simulink library "DriftControllerLibrary"  (R2014a)
settings: Solver=ode45  StartTime=0.0  StopTime=10.0  RelTol=1e-3
values from neighbouring files (symbols this model uses):
  alpha_lookup = alpha_sl:-0.001:-1*alpha_sl    [Fyf_lookup_table.m]
  alpha_prm = 0.9    [InitMap.m]
  beta_prm = 1    [InitMap.m]
  curve_prm = curve_prm.data    [InitMap.m]
  discrete_prm = discrete_prm.data    [InitMap.m]
  errLim_prm = 0.005    [InitMap.m]
  Fyf_lookup_2W = -Cf*tan(alpha_lookup) + Cf^2*(2 - mu_s_assumed_f/mu_p_assumed_f)*abs(tan(alpha_lookup)).*tan(alpha_lookup)/(3*mu_p_assumed_f*Fzf) -      Cf^3*tan(alpha_lookup).^3*(1-2*mu_s_assumed_f/(3*mu_p_assumed_f))/(9*mu_p_assumed_f^2*Fzf^2)    [Fyf_lookup_table.m]
  Fyf_lookup_4W = -(Cf/2)*tan(alpha_lookup) + (Cf/2)^2*(2 - mu_s_assumed_f/mu_p_assumed_f)*abs(tan(alpha_lookup)).*tan(alpha_lookup)/(3*mu_p_assumed_f*(Fzf/2)) -      (Cf/2)^3*tan(alpha_lookup).^3*(1-2*mu_s_assumed_f/(3*mu_p_assumed_f))/(9*mu_p_assumed_f^2*(Fzf/2)^2)    [Fyf_lookup_table.m]
  iterLim_prm = 30    [InitMap.m]
  map_prm = map_prm.data    [InitMap.m]
  numTerms_prm = 10    [InitMap.m]
  seg_prm = seg_prm.data    [InitMap.m]
  Ts = 0.002    [DSC_Control_Analysis.m]    (also in DSC_Control_Analysis_Exp.m; DSC_Speed_Control_Analysis.m; EC_params_nissan.m; Ext_MPCPara.m = SSD.Ts)
  useZ_prm = 0    [InitMap.m]
undefined symbols (not defined in the file or in its folder): ack, axInit, beta_vec, betaDes, betaThreshold, delta_sol, deltaLimits, Feasible, Fxr_sol, FxrEq, Fyf_sat, Fyf_sol, Kbeta, Kr, KUx, KUx_Drift, mu_p_assumed, mu_s_assumed, param, r_vec, rThreshold, sr, steering_limit, tau_DK, tau_DSC, tHold, tLimits, Ux_vec, UxEq, UxLimits, VoltsToTorque, VoltsToTorqueRegen, wc
libraries: DriftControllerLibrary x2, simulink x1
(part 2 of 2)

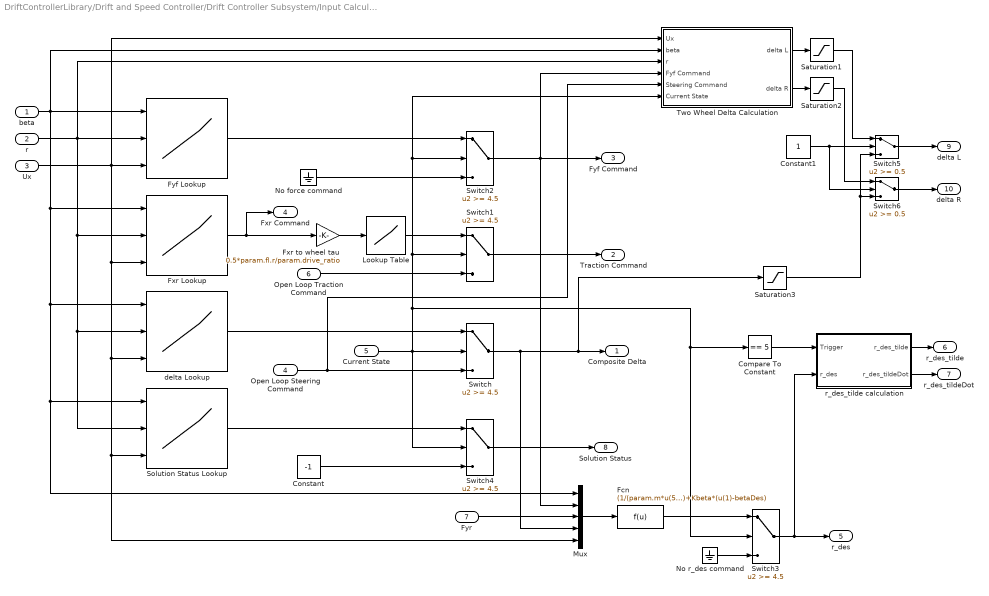
== system DriftControllerLibrary/Drift and Speed Controller/Drift Controller Subsystem/Input Calculation ==
  beta : Inport
  r : Inport  Port=2
  Ux : Inport  Port=3
  Open Loop Steering Command : Inport  Port=4
  Current State : Inport  Port=5
  Open Loop Traction Command : Inport  Port=6
  Fyr : Inport  Port=7
  Compare To Constant : simulink/Logic and Bit Operations/Compare To Constant  relop===  const=5  OutDataTypeStr=uint8  ZeroCross=off
  Constant : Constant  Value=-1
  Constant1 : Constant
  Fcn : Fcn  Expr=(1/(param.m*u(5)))*(u(2)*cos(u(4)) + u(3))+Kbeta*(u(1)-betaDes)
  Fxr Lookup : Lookup_n-D  NumberOfTableDimensions=3  BreakpointsForDimension1=beta_vec  BreakpointsForDimension2=r_vec  BreakpointsForDimension3=Ux_vec  IndexSearchMethod=Evenly spaced points  Table=Fxr_sol  ExtrapMethod=Clip  UseLastTableValue=on  InputSameDT=on
  Fxr to wheel tau : Gain  Gain=0.5*param.fl.r/param.drive_ratio
  Fyf Lookup : Lookup_n-D  NumberOfTableDimensions=3  BreakpointsForDimension1=beta_vec  BreakpointsForDimension2=r_vec  BreakpointsForDimension3=Ux_vec  IndexSearchMethod=Evenly spaced points  Table=Fyf_sol  ExtrapMethod=Clip  UseLastTableValue=on  InputSameDT=on
  Lookup Table : Lookup  InputValues=[-90,0,210]  Table=[1.1,1.95,2.8]  LookUpMeth=Interpolation-Use End Values
  Mux : Mux  Inputs=5
  No force command : Ground
  No r_des command : Ground
  Saturation1 : Saturate  UpperLimit=steering_limit*pi/180  LowerLimit=-steering_limit*pi/180
  Saturation2 : Saturate  UpperLimit=steering_limit*pi/180  LowerLimit=-steering_limit*pi/180
  Saturation3 : Saturate  UpperLimit=steering_limit*pi/180  LowerLimit=-steering_limit*pi/180
  Solution Status Lookup : Lookup_n-D  NumberOfTableDimensions=3  BreakpointsForDimension1=beta_vec  BreakpointsForDimension2=r_vec  BreakpointsForDimension3=Ux_vec  IndexSearchMethod=Evenly spaced points  Table=Feasible  ExtrapMethod=Clip  UseLastTableValue=on  InputSameDT=on
  Switch{,1..4} (5 alike) : Switch  Threshold=4.5
  Switch5 : Switch  Threshold=0.5
  Switch6 : Switch  Threshold=0.5
  Two Wheel Delta Calculation : Subsystem
  delta Lookup : Lookup_n-D  NumberOfTableDimensions=3  BreakpointsForDimension1=beta_vec  BreakpointsForDimension2=r_vec  BreakpointsForDimension3=Ux_vec  IndexSearchMethod=Evenly spaced points  Table=delta_sol  ExtrapMethod=Clip  UseLastTableValue=on  InputSameDT=on
  r_des_tilde calculation : Subsystem
  Composite Delta : Outport
  Traction Command : Outport  Port=2
  Fyf Command : Outport  Port=3
  Fxr Command : Outport  Port=4
  r_des : Outport  Port=5
  r_des_tilde : Outport  Port=6
  r_des_tildeDot : Outport  Port=7
  Solution Status : Outport  Port=8
  delta L : Outport  Port=9
  delta R : Outport  Port=10
  wires:
  Constant1/1 -> Switch6/2, Switch5/2
  Saturation3/1 -> Switch6/3, Switch5/3
  Saturation2/1 -> Switch6/1
  Saturation1/1 -> Switch5/1
  Switch5/1 -> delta L/1
  Switch6/1 -> delta R/1
  delta Lookup/1 -> Switch/1
  Open Loop Steering Command/1 -> Switch/3, Two Wheel Delta Calculation/5(Steering Command)
  Switch/1 -> Saturation3/1, Composite Delta/1, Mux/4
  Fyf Lookup/1 -> Switch2/1
  Open Loop Traction Command/1 -> Switch1/3
  No force command/1 -> Switch2/3
  Fxr Lookup/1 -> Fxr Command/1, Fxr to wheel tau/1
  Switch1/1 -> Traction Command/1
  Switch2/1 -> Fyf Command/1, Mux/2, Two Wheel Delta Calculation/4(Fyf Command)
  Fyr/1 -> Mux/3
  Mux/1 -> Fcn/1
  Current State/1 -> Switch/2, Switch1/2, Switch2/2, Two Wheel Delta Calculation/6(Current State), Switch3/2, Compare To Constant/1, Switch4/2
  Fcn/1 -> Switch3/1
  No r_des command/1 -> Switch3/3
  Switch3/1 -> r_des/1, r_des_tilde calculation/2(r_des)
  Compare To Constant/1 -> r_des_tilde calculation/1(Trigger)
  r_des_tilde calculation/1(r_des_tilde) -> r_des_tilde/1
  r_des_tilde calculation/2(r_des_tildeDot) -> r_des_tildeDot/1
  Solution Status Lookup/1 -> Switch4/1
  Constant/1 -> Switch4/3
  Switch4/1 -> Solution Status/1
  Fxr to wheel tau/1 -> Lookup Table/1
  Lookup Table/1 -> Switch1/1
  beta/1 -> Fyf Lookup/1, Fxr Lookup/1, delta Lookup/1, Solution Status Lookup/1, Mux/1, Two Wheel Delta Calculation/2(beta)
  r/1 -> Fyf Lookup/2, Fxr Lookup/2, delta Lookup/2, Solution Status Lookup/2, Two Wheel Delta Calculation/3(r)
  Ux/1 -> Fyf Lookup/3, Fxr Lookup/3, delta Lookup/3, Solution Status Lookup/3, Mux/5, Two Wheel Delta Calculation/1(Ux)
  Two Wheel Delta Calculation/2(delta R) -> Saturation2/1
  Two Wheel Delta Calculation/1(delta L) -> Saturation1/1

== system DriftControllerLibrary/Drift and Speed Controller/Enable Logic/Delay ==
  In : Inport
  Unit Delay{,1..4} (5 alike) : UnitDelay  SampleTime=Ts
  Out : Outport
  wires:
  In/1 -> Unit Delay/1
  Unit Delay/1 -> Unit Delay1/1
  Unit Delay1/1 -> Unit Delay2/1
  Unit Delay2/1 -> Unit Delay3/1
  Unit Delay3/1 -> Unit Delay4/1
  Unit Delay4/1 -> Out/1

== system DriftControllerLibrary/Drift and Speed Controller/Enable Logic/Latch1 ==
  In1 : Inport
  Trigger : TriggerPort
  Out1 : Outport  InitialOutput=0
  wires:
  In1/1 -> Out1/1

== system DriftControllerLibrary/Driftkeeping/Driftkeeping Subsystem/Map-Matching SCACS2 ==
  GPS Vehicle State : Inport
  Enable : Inport  Port=2
  Bus Creator : BusCreator  Inputs=6
  Bus Selector : BusSelector  OutputSignals=Pos E,Pos N,Yaw Angle,Vx
  Constant1 : Constant  Value=pi/2  SampleTime=Ts
  Ground : Ground
  SCACS Map-Matching : Subsystem
  Sum : Sum  Inputs=|++
  SCACS : Outport
  wires:
  Bus Selector/4 -> SCACS Map-Matching/5(vx_cg)  "<Vx>"
  Bus Selector/3 -> Sum/1  "<Yaw Angle>"
  Ground/1 -> SCACS Map-Matching/3(posU)
  Enable/1 -> SCACS Map-Matching/6(enable)
  Bus Creator/1 -> SCACS/1
  Bus Selector/2 -> SCACS Map-Matching/2(posN)  "<Pos N>"
  Bus Selector/1 -> SCACS Map-Matching/1(posE)  "<Pos E>"
  GPS Vehicle State/1 -> Bus Selector/1
  SCACS Map-Matching/1(matchOut) -> Bus Creator/1  "matchOut"
  SCACS Map-Matching/2(curOut) -> Bus Creator/2  "curOut"
  SCACS Map-Matching/3(nxtOut) -> Bus Creator/3  "nxtOut"
  SCACS Map-Matching/4(twoOut) -> Bus Creator/4  "twoOut"
  SCACS Map-Matching/5(thrOut) -> Bus Creator/5  "thrOut"
  Constant1/1 -> Sum/2
  Sum/1 -> SCACS Map-Matching/4(yaw)
  SCACS Map-Matching/6(debugOut) -> Bus Creator/6  "debugOut"

== system DriftControllerLibrary/Driftkeeping/Driftkeeping Subsystem/Single Wheel Delta Calculation ==
  Ux : Inport
  Uy : Inport  Port=2
  r : Inport  Port=3
  Fyf Command : Inport  Port=4
  Steering Command : Inport  Port=5
  Current State : Inport  Port=6
  Lookup Table : Lookup  InputValues=Fyf_lookup_2W  Table=alpha_lookup  LookUpMeth=Interpolation-Use End Values
  Mux1 : Mux  Inputs=3
  "Slip Angle " : Fcn  Expr=atan2(u[2] + param.a*u[3], u[1])*(u[1] >= 0.5)
  Sum : Sum  Inputs=+-|
  Switch : Switch  Threshold=1.5
  Composite Delta : Outport
  wires:
  Mux1/1 -> "Slip Angle "/1
  Lookup Table/1 -> Sum/2
  "Slip Angle "/1 -> Sum/1
  Sum/1 -> Switch/1
  Steering Command/1 -> Switch/3
  Current State/1 -> Switch/2
  Fyf Command/1 -> Lookup Table/1
  Ux/1 -> Mux1/1
  Uy/1 -> Mux1/2
  r/1 -> Mux1/3
  Switch/1 -> Composite Delta/1

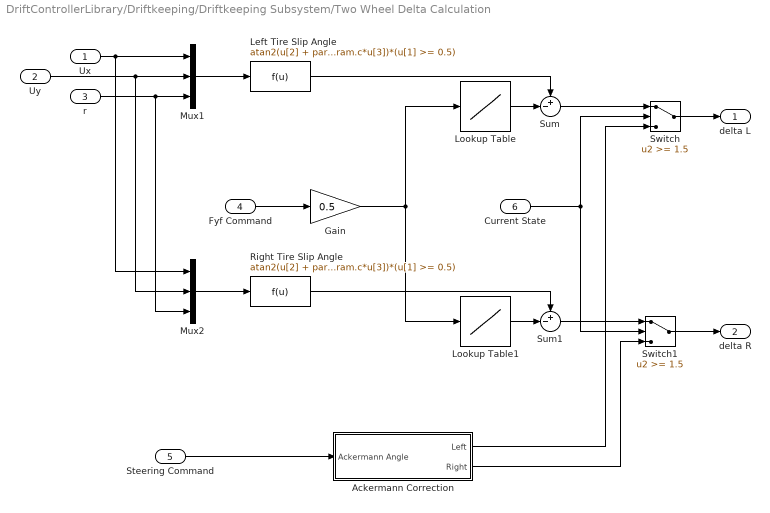
== system DriftControllerLibrary/Driftkeeping/Driftkeeping Subsystem/Two Wheel Delta Calculation ==
  Ux : Inport
  Uy : Inport  Port=2
  r : Inport  Port=3
  Fyf Command : Inport  Port=4
  Steering Command : Inport  Port=5
  Current State : Inport  Port=6
  Ackermann Correction : Subsystem
  Gain : Gain  Gain=0.5
  Left Tire Slip Angle : Fcn  Expr=atan2(u[2] + param.a*u[3], u[1]-param.c*u[3])*(u[1] >= 0.5)
  Lookup Table : Lookup  InputValues=Fyf_lookup_4W  Table=alpha_lookup  LookUpMeth=Interpolation-Use End Values
  Lookup Table1 : Lookup  InputValues=Fyf_lookup_4W  Table=alpha_lookup  LookUpMeth=Interpolation-Use End Values
  Mux1 : Mux  Inputs=3
  Mux2 : Mux  Inputs=3
  Right Tire Slip Angle : Fcn  Expr=atan2(u[2] + param.a*u[3], u[1]+param.c*u[3])*(u[1] >= 0.5)
  Sum : Sum  Inputs=+-|
  Sum1 : Sum  Inputs=+-|
  Switch : Switch  Threshold=1.5
  Switch1 : Switch  Threshold=1.5
  delta L : Outport
  delta R : Outport  Port=2
  wires:
  Mux1/1 -> Left Tire Slip Angle/1
  Lookup Table/1 -> Sum/2
  Left Tire Slip Angle/1 -> Sum/1
  Sum/1 -> Switch/1
  Ux/1 -> Mux1/1, Mux2/1
  Uy/1 -> Mux1/2, Mux2/2
  r/1 -> Mux1/3, Mux2/3
  Switch/1 -> delta L/1
  Mux2/1 -> Right Tire Slip Angle/1
  Fyf Command/1 -> Gain/1
  Gain/1 -> Lookup Table/1, Lookup Table1/1
  Lookup Table1/1 -> Sum1/2
  Right Tire Slip Angle/1 -> Sum1/1
  Switch1/1 -> delta R/1
  Sum1/1 -> Switch1/1
  Current State/1 -> Switch/2, Switch1/2
  Steering Command/1 -> Ackermann Correction/1(Ackermann Angle)
  Ackermann Correction/1(Left) -> Switch/3
  Ackermann Correction/2(Right) -> Switch1/3

== system DriftControllerLibrary/Driftkeeping/Enable Logic/Delay ==
  In : Inport
  Unit Delay{,1..4} (5 alike) : UnitDelay  SampleTime=Ts
  Out : Outport
  wires:
  In/1 -> Unit Delay/1
  Unit Delay/1 -> Unit Delay1/1
  Unit Delay1/1 -> Unit Delay2/1
  Unit Delay2/1 -> Unit Delay3/1
  Unit Delay3/1 -> Unit Delay4/1
  Unit Delay4/1 -> Out/1

== system DriftControllerLibrary/Driftkeeping/Enable Logic/Latch1 ==
  In1 : Inport
  Trigger : TriggerPort
  Out1 : Outport  InitialOutput=0
  wires:
  In1/1 -> Out1/1

== system DriftControllerLibrary/SSC Drift Controller/Enable Logic/Delay ==
  In : Inport
  Unit Delay{,1..4} (5 alike) : UnitDelay  SampleTime=Ts
  Out : Outport
  wires:
  In/1 -> Unit Delay/1
  Unit Delay/1 -> Unit Delay1/1
  Unit Delay1/1 -> Unit Delay2/1
  Unit Delay2/1 -> Unit Delay3/1
  Unit Delay3/1 -> Unit Delay4/1
  Unit Delay4/1 -> Out/1

== system DriftControllerLibrary/SSC Drift Controller/Enable Logic/Latch1 ==
  In1 : Inport
  Trigger : TriggerPort
  Out1 : Outport  InitialOutput=0
  wires:
  In1/1 -> Out1/1

== system DriftControllerLibrary/Simplified Drift Control/Drift Controller Subsystem/Single Wheel Delta Calculation ==
  Ux : Inport
  Uy : Inport  Port=2
  r : Inport  Port=3
  Fyf Command : Inport  Port=4
  Steering Command : Inport  Port=5
  Current State : Inport  Port=6
  Lookup Table : Lookup  InputValues=Fyf_lookup_2W  Table=alpha_lookup  LookUpMeth=Interpolation-Use End Values
  Mux1 : Mux  Inputs=3
  "Slip Angle " : Fcn  Expr=atan2(u[2] + param.a*u[3], u[1])*(u[1] >= 0.5)
  Sum : Sum  Inputs=+-|
  Switch : Switch  Threshold=4.5
  Composite Delta : Outport
  wires:
  Switch/1 -> Composite Delta/1
  r/1 -> Mux1/3
  Uy/1 -> Mux1/2
  Ux/1 -> Mux1/1
  Fyf Command/1 -> Lookup Table/1
  Current State/1 -> Switch/2
  Steering Command/1 -> Switch/3
  Sum/1 -> Switch/1
  "Slip Angle "/1 -> Sum/1
  Lookup Table/1 -> Sum/2
  Mux1/1 -> "Slip Angle "/1

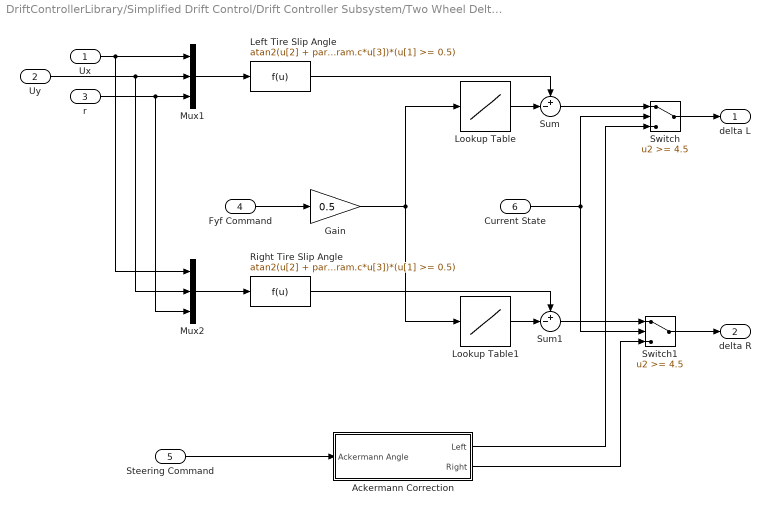
== system DriftControllerLibrary/Simplified Drift Control/Drift Controller Subsystem/Two Wheel Delta Calculation ==
  Ux : Inport
  Uy : Inport  Port=2
  r : Inport  Port=3
  Fyf Command : Inport  Port=4
  Steering Command : Inport  Port=5
  Current State : Inport  Port=6
  Ackermann Correction : Subsystem
  Gain : Gain  Gain=0.5
  Left Tire Slip Angle : Fcn  Expr=atan2(u[2] + param.a*u[3], u[1]-param.c*u[3])*(u[1] >= 0.5)
  Lookup Table : Lookup  InputValues=Fyf_lookup_4W  Table=alpha_lookup  LookUpMeth=Interpolation-Use End Values
  Lookup Table1 : Lookup  InputValues=Fyf_lookup_4W  Table=alpha_lookup  LookUpMeth=Interpolation-Use End Values
  Mux1 : Mux  Inputs=3
  Mux2 : Mux  Inputs=3
  Right Tire Slip Angle : Fcn  Expr=atan2(u[2] + param.a*u[3], u[1]+param.c*u[3])*(u[1] >= 0.5)
  Sum : Sum  Inputs=+-|
  Sum1 : Sum  Inputs=+-|
  Switch : Switch  Threshold=4.5
  Switch1 : Switch  Threshold=4.5
  delta L : Outport
  delta R : Outport  Port=2
  wires:
  Ackermann Correction/2(Right) -> Switch1/3
  Ackermann Correction/1(Left) -> Switch/3
  Steering Command/1 -> Ackermann Correction/1(Ackermann Angle)
  Current State/1 -> Switch1/2, Switch/2
  Sum1/1 -> Switch1/1
  Switch1/1 -> delta R/1
  Right Tire Slip Angle/1 -> Sum1/1
  Lookup Table1/1 -> Sum1/2
  Gain/1 -> Lookup Table1/1, Lookup Table/1
  Fyf Command/1 -> Gain/1
  Mux2/1 -> Right Tire Slip Angle/1
  Switch/1 -> delta L/1
  r/1 -> Mux2/3, Mux1/3
  Uy/1 -> Mux2/2, Mux1/2
  Ux/1 -> Mux2/1, Mux1/1
  Sum/1 -> Switch/1
  Left Tire Slip Angle/1 -> Sum/1
  Lookup Table/1 -> Sum/2
  Mux1/1 -> Left Tire Slip Angle/1

== system DriftControllerLibrary/Simplified Drift Control/Enable Logic/Delay ==
  In : Inport
  Unit Delay{,1..4} (5 alike) : UnitDelay  SampleTime=Ts
  Out : Outport
  wires:
  Unit Delay4/1 -> Out/1
  Unit Delay3/1 -> Unit Delay4/1
  Unit Delay2/1 -> Unit Delay3/1
  Unit Delay1/1 -> Unit Delay2/1
  Unit Delay/1 -> Unit Delay1/1
  In/1 -> Unit Delay/1

== system DriftControllerLibrary/Simplified Drift Control/Enable Logic/Latch1 ==
  In1 : Inport
  Trigger : TriggerPort
  Out1 : Outport  InitialOutput=0
  wires:
  In1/1 -> Out1/1

== system DriftControllerLibrary/Drift Control Block/Drift Controller Subsystem/Two Wheel Delta Calculation/Ackermann Correction ==
  Ackermann Angle : Inport
  left ackermann ideal correction angle : Fcn  Expr=u/(1-u*ack*param.tw/2/(param.a+param.b))
  right ackermann ideal correction angle : Fcn  Expr=u/(1+u*ack*param.tw/2/(param.a+param.b))
  Left : Outport
  Right : Outport  Port=2
  wires:
  left ackermann ideal correction angle/1 -> Left/1
  right ackermann ideal correction angle/1 -> Right/1
  Ackermann Angle/1 -> left ackermann ideal correction angle/1, right ackermann ideal correction angle/1

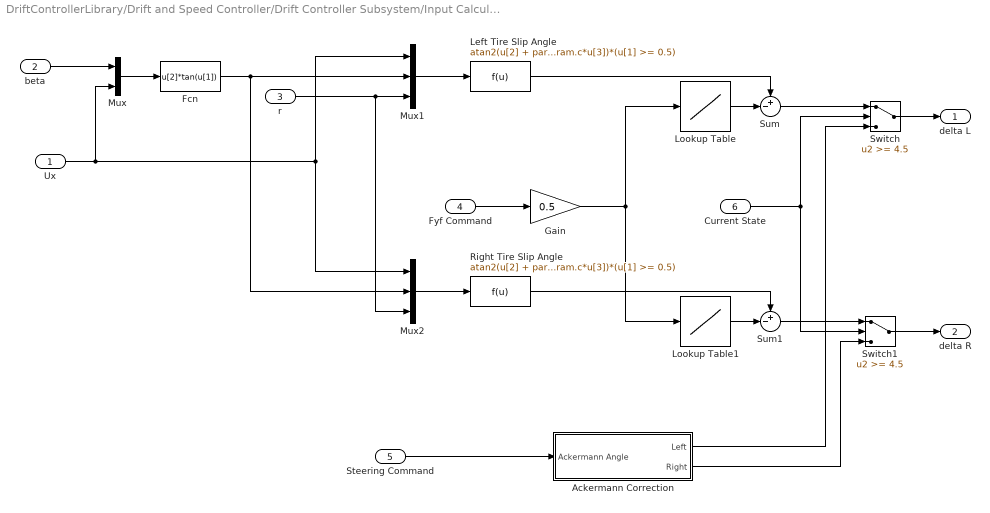
== system DriftControllerLibrary/Drift and Speed Controller/Drift Controller Subsystem/Input Calculation/Two Wheel Delta Calculation ==
  Ux : Inport
  beta : Inport  Port=2
  r : Inport  Port=3
  Fyf Command : Inport  Port=4
  Steering Command : Inport  Port=5
  Current State : Inport  Port=6
  Ackermann Correction : Subsystem
  Fcn : Fcn  Expr=u[2]*tan(u[1])
  Gain : Gain  Gain=0.5
  Left Tire Slip Angle : Fcn  Expr=atan2(u[2] + param.a*u[3], u[1]-param.c*u[3])*(u[1] >= 0.5)
  Lookup Table : Lookup  InputValues=Fyf_lookup_4W  Table=alpha_lookup  LookUpMeth=Interpolation-Use End Values
  Lookup Table1 : Lookup  InputValues=Fyf_lookup_4W  Table=alpha_lookup  LookUpMeth=Interpolation-Use End Values
  Mux : Mux  Inputs=2
  Mux1 : Mux  Inputs=3
  Mux2 : Mux  Inputs=3
  Right Tire Slip Angle : Fcn  Expr=atan2(u[2] + param.a*u[3], u[1]+param.c*u[3])*(u[1] >= 0.5)
  Sum : Sum  Inputs=+-|
  Sum1 : Sum  Inputs=+-|
  Switch : Switch  Threshold=4.5
  Switch1 : Switch  Threshold=4.5
  delta L : Outport
  delta R : Outport  Port=2
  wires:
  Ackermann Correction/2(Right) -> Switch1/3
  Ackermann Correction/1(Left) -> Switch/3
  Steering Command/1 -> Ackermann Correction/1(Ackermann Angle)
  Current State/1 -> Switch1/2, Switch/2
  Sum1/1 -> Switch1/1
  Switch1/1 -> delta R/1
  Right Tire Slip Angle/1 -> Sum1/1
  Lookup Table1/1 -> Sum1/2
  Gain/1 -> Lookup Table1/1, Lookup Table/1
  Fyf Command/1 -> Gain/1
  Mux2/1 -> Right Tire Slip Angle/1
  Switch/1 -> delta L/1
  r/1 -> Mux2/3, Mux1/3
  Sum/1 -> Switch/1
  Left Tire Slip Angle/1 -> Sum/1
  Lookup Table/1 -> Sum/2
  Mux1/1 -> Left Tire Slip Angle/1
  Ux/1 -> Mux/2, Mux2/1, Mux1/1
  beta/1 -> Mux/1
  Mux/1 -> Fcn/1
  Fcn/1 -> Mux1/2, Mux2/2

== system DriftControllerLibrary/Drift and Speed Controller/Drift Controller Subsystem/Input Calculation/r_des_tilde calculation ==
  Trigger : Inport
  r_des : Inport  Port=2
  Clock : Clock
  Discrete Zero-Pole2 : DiscreteZeroPole  Zeros=[]  Poles=[exp(-Ts/tau_DSC)]  Gain=1-exp(-Ts/tau_DSC)  SampleTime=Ts
  Fcn : Fcn  Expr=u(1)*exp(-(u(3)-u(2))/tau_DSC)
  Fcn1 : Fcn  Expr=(1/tau_DSC)*(u(2)-u(1))
  Mux : Mux  Inputs=3
  Mux1 : Mux  Inputs=2
  Product : Product  RndMeth=Zero
  Scope : Scope
  Sum : Sum  Inputs=|++
  Triggered Subsystem : Subsystem  TreatAsAtomicUnit=on
  r_des_tilde : Outport
  r_des_tildeDot : Outport  Port=2
  wires:
  Fcn/1 -> Scope/1, Sum/1
  Trigger/1 -> Triggered Subsystem/Trigger, Product/1
  r_des/1 -> Triggered Subsystem/1(r_des), Discrete Zero-Pole2/1, Mux1/2
  Clock/1 -> Triggered Subsystem/2(t), Mux/3
  Triggered Subsystem/1(r_des0) -> Mux/1
  Triggered Subsystem/2(t_start) -> Mux/2
  Mux/1 -> Fcn/1
  Discrete Zero-Pole2/1 -> Sum/2
  Sum/1 -> Product/2
  Product/1 -> r_des_tilde/1, Mux1/1
  Mux1/1 -> Fcn1/1
  Fcn1/1 -> r_des_tildeDot/1

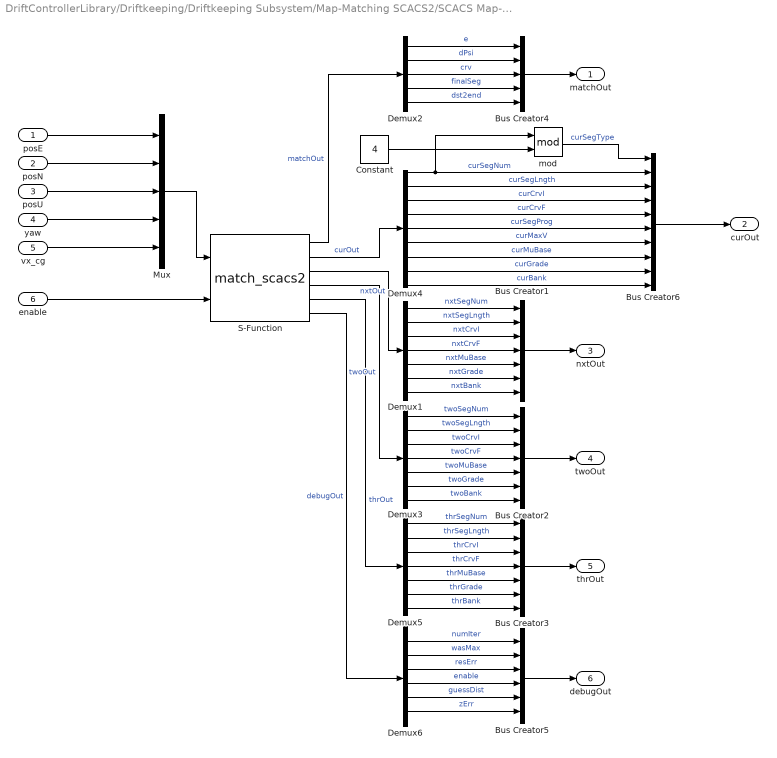
== system DriftControllerLibrary/Driftkeeping/Driftkeeping Subsystem/Map-Matching SCACS2/SCACS Map-Matching ==
  posE : Inport
  posN : Inport  Port=2
  posU : Inport  Port=3
  yaw : Inport  Port=4
  vx_cg : Inport  Port=5
  enable : Inport  Port=6
  Bus Creator1 : BusCreator  Inputs=7
  Bus Creator2 : BusCreator  Inputs=7
  Bus Creator3 : BusCreator  Inputs=7
  Bus Creator4 : BusCreator  Inputs=5
  Bus Creator5 : BusCreator  Inputs=6
  Bus Creator6 : BusCreator  Inputs=10
  Constant : Constant  Value=4
  Demux1 : Demux  Outputs=7
  Demux2 : Demux  Outputs=5
  Demux3 : Demux  Outputs=7
  Demux4 : Demux  Outputs=9
  Demux5 : Demux  Outputs=7
  Demux6 : Demux  Outputs=6
  Mux : Mux  Inputs=5
  S-Function : S-Function  FunctionName=match_scacs2  Parameters=errLim_prm,iterLim_prm,alpha_prm,numTerms_prm,useZ_prm,beta_prm,map_prm,curve_prm,seg_prm,discrete_prm  EnableBusSupport=off
      mask init:
      | InitMap
  mod : Math  Operator=mod  SaturateOnIntegerOverflow=on
  matchOut : Outport
  curOut : Outport  Port=2
  nxtOut : Outport  Port=3
  twoOut : Outport  Port=4
  thrOut : Outport  Port=5
  debugOut : Outport  Port=6
  wires:
  enable/1 -> S-Function/2
  vx_cg/1 -> Mux/5
  yaw/1 -> Mux/4
  posU/1 -> Mux/3
  Demux2/2 -> Bus Creator4/2  "dPsi"
  S-Function/2 -> Demux4/1  "curOut"
  Bus Creator5/1 -> debugOut/1
  Bus Creator3/1 -> thrOut/1
  Bus Creator2/1 -> twoOut/1
  Bus Creator1/1 -> nxtOut/1
  Bus Creator4/1 -> matchOut/1
  Demux4/9 -> Bus Creator6/10  "curBank"
  Demux4/8 -> Bus Creator6/9  "curGrade"
  Demux4/7 -> Bus Creator6/8  "curMuBase"
  Demux4/6 -> Bus Creator6/7  "curMaxV"
  Demux4/5 -> Bus Creator6/6  "curSegProg"
  Demux4/4 -> Bus Creator6/5  "curCrvF"
  Demux4/3 -> Bus Creator6/4  "curCrvI"
  Demux4/2 -> Bus Creator6/3  "curSegLngth"
  Demux4/1 -> Bus Creator6/2, mod/1  "curSegNum"
  Demux2/5 -> Bus Creator4/5  "dst2end"
  Demux2/4 -> Bus Creator4/4  "finalSeg"
  Demux2/3 -> Bus Creator4/3  "crv"
  Demux2/1 -> Bus Creator4/1  "e"
  Demux6/6 -> Bus Creator5/6  "zErr"
  Demux6/5 -> Bus Creator5/5  "guessDist"
  Demux6/4 -> Bus Creator5/4  "enable"
  Demux6/3 -> Bus Creator5/3  "resErr"
  Demux6/2 -> Bus Creator5/2  "wasMax"
  Demux6/1 -> Bus Creator5/1  "numIter"
  Demux5/7 -> Bus Creator3/7  "thrBank"
  Demux5/6 -> Bus Creator3/6  "thrGrade"
  Demux5/5 -> Bus Creator3/5  "thrMuBase"
  Demux5/4 -> Bus Creator3/4  "thrCrvF"
  Demux5/3 -> Bus Creator3/3  "thrCrvI"
  Demux5/2 -> Bus Creator3/2  "thrSegLngth"
  Demux5/1 -> Bus Creator3/1  "thrSegNum"
  Demux3/7 -> Bus Creator2/7  "twoBank"
  Demux3/6 -> Bus Creator2/6  "twoGrade"
  Demux3/5 -> Bus Creator2/5  "twoMuBase"
  Demux3/4 -> Bus Creator2/4  "twoCrvF"
  Demux3/3 -> Bus Creator2/3  "twoCrvI"
  Demux3/2 -> Bus Creator2/2  "twoSegLngth"
  Demux3/1 -> Bus Creator2/1  "twoSegNum"
  Demux1/7 -> Bus Creator1/7  "nxtBank"
  Demux1/6 -> Bus Creator1/6  "nxtGrade"
  Demux1/5 -> Bus Creator1/5  "nxtMuBase"
  Demux1/4 -> Bus Creator1/4  "nxtCrvF"
  Demux1/3 -> Bus Creator1/3  "nxtCrvI"
  Demux1/2 -> Bus Creator1/2  "nxtSegLngth"
  Demux1/1 -> Bus Creator1/1  "nxtSegNum"
  S-Function/5 -> Demux5/1  "thrOut"
  posN/1 -> Mux/2
  posE/1 -> Mux/1
  S-Function/3 -> Demux1/1  "nxtOut"
  S-Function/1 -> Demux2/1  "matchOut"
  S-Function/4 -> Demux3/1  "twoOut"
  Mux/1 -> S-Function/1
  S-Function/6 -> Demux6/1  "debugOut"
  Constant/1 -> mod/2
  mod/1 -> Bus Creator6/1  "curSegType"
  Bus Creator6/1 -> curOut/1

== system DriftControllerLibrary/Driftkeeping/Driftkeeping Subsystem/Two Wheel Delta Calculation/Ackermann Correction ==
  Ackermann Angle : Inport
  left ackermann ideal correction angle : Fcn  Expr=u/(1-u*ack*param.tw/2/(param.a+param.b))
  right ackermann ideal correction angle : Fcn  Expr=u/(1+u*ack*param.tw/2/(param.a+param.b))
  Left : Outport
  Right : Outport  Port=2
  wires:
  Ackermann Angle/1 -> right ackermann ideal correction angle/1, left ackermann ideal correction angle/1
  right ackermann ideal correction angle/1 -> Right/1
  left ackermann ideal correction angle/1 -> Left/1

== system DriftControllerLibrary/Simplified Drift Control/Drift Controller Subsystem/Two Wheel Delta Calculation/Ackermann Correction ==
  Ackermann Angle : Inport
  left ackermann ideal correction angle : Fcn  Expr=u/(1-u*ack*param.tw/2/(param.a+param.b))
  right ackermann ideal correction angle : Fcn  Expr=u/(1+u*ack*param.tw/2/(param.a+param.b))
  Left : Outport
  Right : Outport  Port=2
  wires:
  left ackermann ideal correction angle/1 -> Left/1
  right ackermann ideal correction angle/1 -> Right/1
  Ackermann Angle/1 -> left ackermann ideal correction angle/1, right ackermann ideal correction angle/1

== system DriftControllerLibrary/Drift and Speed Controller/Drift Controller Subsystem/Input Calculation/Two Wheel Delta Calculation/Ackermann Correction ==
  Ackermann Angle : Inport
  left ackermann ideal correction angle : Fcn  Expr=u/(1-u*ack*param.tw/2/(param.a+param.b))
  right ackermann ideal correction angle : Fcn  Expr=u/(1+u*ack*param.tw/2/(param.a+param.b))
  Left : Outport
  Right : Outport  Port=2
  wires:
  left ackermann ideal correction angle/1 -> Left/1
  right ackermann ideal correction angle/1 -> Right/1
  Ackermann Angle/1 -> left ackermann ideal correction angle/1, right ackermann ideal correction angle/1

== system DriftControllerLibrary/Drift and Speed Controller/Drift Controller Subsystem/Input Calculation/r_des_tilde calculation/Triggered Subsystem ==
  r_des : Inport
  t : Inport  Port=2
  Trigger : TriggerPort
  r_des0 : Outport
  t_start : Outport  Port=2
  wires:
  r_des/1 -> r_des0/1
  t/1 -> t_start/1
